simulink model "clarke"  (R2023a)
settings: Solver=VariableStepAuto  StartTime=0.0  StopTime=10.0  RelTol=1e-3
values from neighbouring files (symbols this model uses):
  k = 1    [init_value.m]
settings Model: Creator=11048  LastModifiedBy=11048

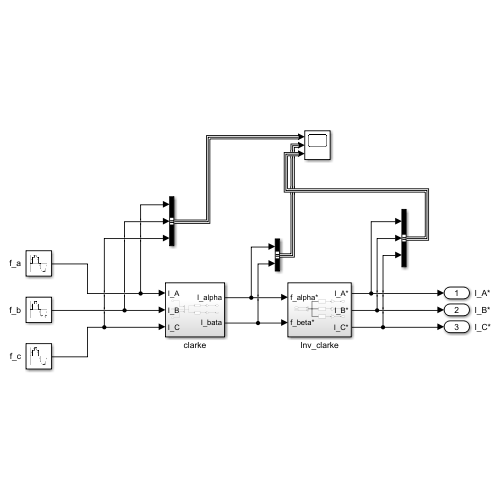
[thumbnail: Simulink's stored preview of the top-level diagram]
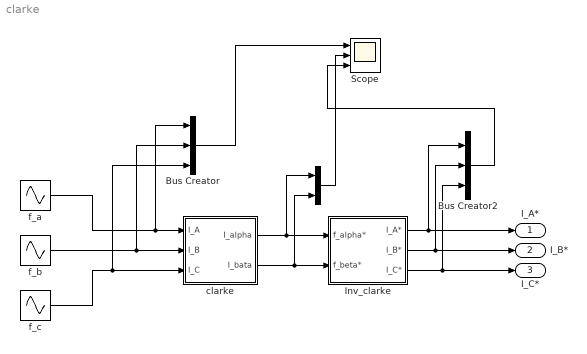
== system clarke ==
  " " : BusCreator  Inputs=2
  Bus Creator : BusCreator  Inputs=3
  Bus Creator2 : BusCreator  Inputs=3
  Inv_clarke : Subsystem
  Scope : Scope  NumInputPorts=3
  clarke : Subsystem
  f_a : Sin  Frequency=2*pi*50  SampleTime=0.00001
  f_b : Sin  Frequency=2*pi*50  Phase=-pi*2/3  SampleTime=0.00001
  f_c : Sin  Frequency=2*pi*50  Phase=pi*2/3  SampleTime=0.00001
  I_A* : Outport
  I_B* : Outport  Port=2
  I_C* : Outport  Port=3
  wires:
  Inv_clarke/1(I_A*) -> I_A*/1, Bus Creator2/1
  Inv_clarke/2(I_B*) -> I_B*/1, Bus Creator2/2
  Inv_clarke/3(I_C*) -> I_C*/1, Bus Creator2/3
  clarke/1(I_alpha) -> " "/1, Inv_clarke/1(f_alpha*)
  clarke/2(I_bata) -> Inv_clarke/2(f_beta*), " "/2
  f_a/1 -> Bus Creator/1, clarke/1(I_A)
  f_b/1 -> Bus Creator/2, clarke/2(I_B)
  f_c/1 -> Bus Creator/3, clarke/3(I_C)
  Bus Creator/1 -> Scope/1
  " "/1 -> Scope/2
  Bus Creator2/1 -> Scope/3

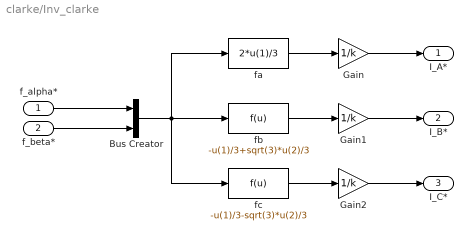
== system clarke/Inv_clarke ==
  f_alpha* : Inport
  f_beta* : Inport  Port=2
  Bus Creator : BusCreator  Inputs=2
  Gain : Gain  Gain=1/k
  Gain1 : Gain  Gain=1/k
  Gain2 : Gain  Gain=1/k
  fa : Fcn  Expr=2*u(1)/3
  fb : Fcn  Expr=-u(1)/3+sqrt(3)*u(2)/3
  fc : Fcn  Expr=-u(1)/3-sqrt(3)*u(2)/3
  I_A* : Outport
  I_B* : Outport  Port=2
  I_C* : Outport  Port=3
  wires:
  Bus Creator/1 -> fc/1, fb/1, fa/1
  f_alpha*/1 -> Bus Creator/1
  f_beta*/1 -> Bus Creator/2
  fa/1 -> Gain/1
  Gain/1 -> I_A*/1
  fb/1 -> Gain1/1
  Gain1/1 -> I_B*/1
  fc/1 -> Gain2/1
  Gain2/1 -> I_C*/1

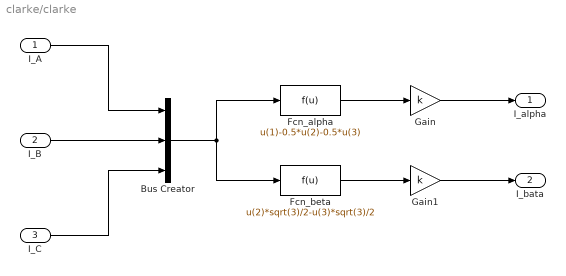
== system clarke/clarke ==
  I_A : Inport
  I_B : Inport  Port=2
  I_C : Inport  Port=3
  Bus Creator : BusCreator  Inputs=3
  Fcn_alpha : Fcn  Expr=u(1)-0.5*u(2)-0.5*u(3)
  Fcn_beta : Fcn  Expr=u(2)*sqrt(3)/2-u(3)*sqrt(3)/2
  Gain : Gain  Gain=k
  Gain1 : Gain  Gain=k
  I_alpha : Outport
  I_bata : Outport  Port=2
  wires:
  Bus Creator/1 -> Fcn_beta/1, Fcn_alpha/1
  I_A/1 -> Bus Creator/1
  I_C/1 -> Bus Creator/3
  I_B/1 -> Bus Creator/2
  Fcn_alpha/1 -> Gain/1
  Gain/1 -> I_alpha/1
  Fcn_beta/1 -> Gain1/1
  Gain1/1 -> I_bata/1
